simulink model "planta"  (Simulink 9.2)
settings: Solver=ode45  StartTime=0.0  StopTime=100  RelTol=1e-3  EnableMultiTasking=on
libraries: fuzblock x1
settings Model: Creator=juan  LastModifiedBy=Rocío  ExtModeAutoUpdateStatusClock=off
settings OptimizationCC: InitFltsAndDblsToZero=on
settings DebuggingCC: SaveWithParameterizedLinksMsg=none  SignalResolutionControl=TryResolveAllWithWarning  SolverPrmCheckMsg=warning  StateNameClashWarn=none
settings SFSimCC: SimUseLocalCustomCode=on
settings RTWCC: RTWUseLocalCustomCode=on
settings GRTTargetCC: TargetFcnLib=ansi_tfl_tmw.mat  GeneratePreprocessorConditionals=Use local settings
settings ConfigComp: CovExternalEMLEnable=on

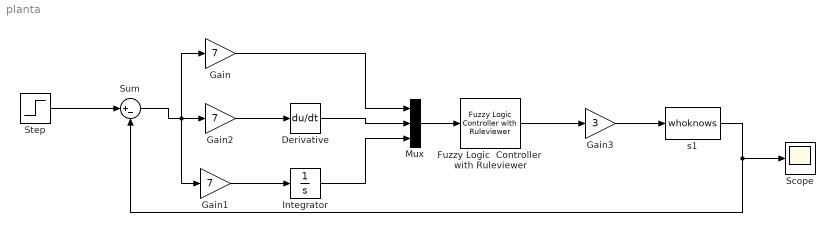
== system planta ==
  Derivative : Derivative  CoefficientInTFapproximation=1
  Fuzzy Logic  Controller  with Ruleviewer : fuzblock/Fuzzy Logic  Controller  with Ruleviewer  fismatrix=Fuzzy3  Ts=2
  Gain : Gain  Gain=7
  Gain1 : Gain  Gain=7
  Gain2 : Gain  Gain=7
  Gain3 : Gain  Gain=3
  Integrator : Integrator
  Mux : Mux  Inputs=3
  Scope : Scope
  Step : Step  SampleTime=0
  Sum : Sum  Inputs=|+-
  s1 : M-S-Function  FunctionName=whoknows  Parameters=L, P1, P2, T, R  mask{L=7, P1=0, P2=4, T=2, R=0}
      mask prompts: L "Laboratorio"; P1 "Primer digito del Puesto"; P2 "Segundo digito del Puesto"; T "Tipo de Planta"; R "Ruido"
      mask Display: disp('Sistema')
  wires:
  Step/1 -> Sum/1
  Sum/1 -> Gain1/1, Gain/1, Gain2/1
  Gain2/1 -> Derivative/1
  Gain1/1 -> Integrator/1
  Integrator/1 -> Mux/3
  Derivative/1 -> Mux/2
  Gain/1 -> Mux/1
  Gain3/1 -> s1/1
  Fuzzy Logic  Controller  with Ruleviewer/1 -> Gain3/1
  Mux/1 -> Fuzzy Logic  Controller  with Ruleviewer/1
  s1/1 -> Sum/2, Scope/1
